simulink model "lr4"  (R2022a)
settings: Solver=FixedStepAuto  StartTime=0.0  StopTime=inf  FixedStep=1e-2  RelTol=1e-3
libraries: instrumentseriallib x3
settings Model: Creator=User  LastModifiedBy=User

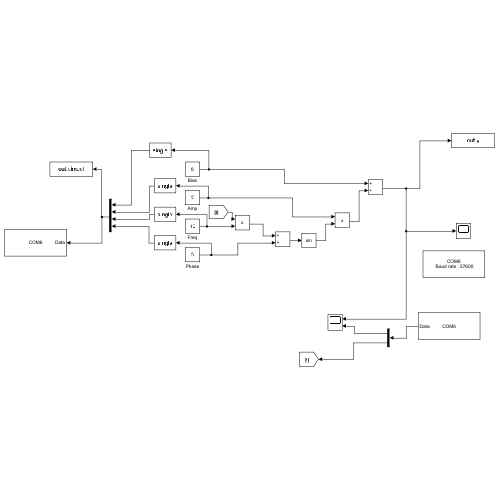
[thumbnail: Simulink's stored preview of the top-level diagram]
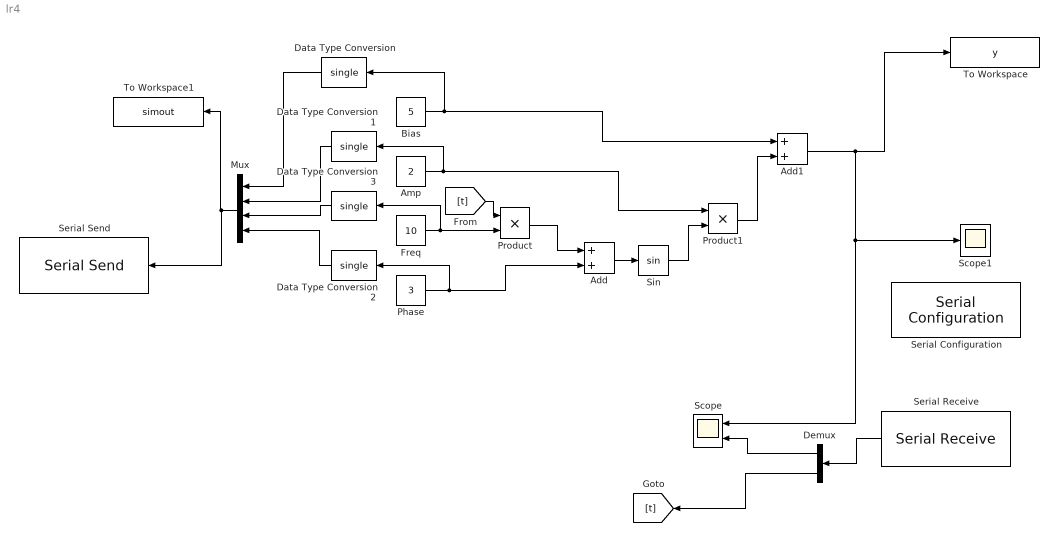
== system lr4 ==
  Add : Sum
  Add1 : Sum
  Amp : Constant  Value=2  OutDataTypeStr=int8
  Bias : Constant  Value=5  OutDataTypeStr=int8
  Data Type Conversion{,1..3} (4 alike) : DataTypeConversion  OutDataTypeStr=single  SaturateOnIntegerOverflow=off  RndMeth=Floor
  Demux : Demux  Outputs=2
  Freq : Constant  Value=10  OutDataTypeStr=int8
  Mux : Mux
  Phase : Constant  Value=3  OutDataTypeStr=int8
  Product : Product
  Product1 : Product
  Scope : Scope  NumInputPorts=2
  Scope1 : Scope
  Serial Configuration : instrumentseriallib/Serial Configuration  Priority=-200000  PortSel=COM6  Port=COM6  ComPort=COM6  BaudRate=57600  DataBits=8  Parity=none  StopBits=1  ByteOrder=little-endian  FlowControl=none  Timeout=10  SimulateUsing=Interpreted execution  BlockInModel=on  aMode=1
      settings: SourceProductBaseCode=OT,IC,MT
  Serial Receive : instrumentseriallib/Serial Receive  Priority=1  PortSel=COM6  Port=COM6  ComPort=COM6  DataType=single  SaveDataType=uint8  ToggleHeader=on  Header='rrrr'  ToggleTerminator=on  Terminator=Custom terminator  CustomTerminator='nnnn'  InputFormat=Row major  ToggleDataSize=on  DataSize=[1 2]  EnableBlockingMode=on  ActionDataUnavailable=Output custom value  ActionWhenDataUnavailable=Output custom value  CustomValue=-1  SampleTime=0.01  SimulateUsing=Interpreted execution  BlockInModel=on  aMode=1
      settings: SourceProductBaseCode=OT,IC,MT
  Serial Send : instrumentseriallib/Serial Send  Priority=1  PortSel=COM6  Port=COM6  ComPort=COM6  Header='rrrr'  Terminator=Custom terminator  CustomTerminator='nnnn'  EnableBlockingMode=on  SimulateUsing=Interpreted execution  BlockInModel=on  aMode=1
      settings: SourceProductBaseCode=OT,IC,MT
  Sin : Trigonometry
  To Workspace : ToWorkspace  VariableName=y  SaveFormat=Timeseries  SampleTime=-1
  To Workspace1 : ToWorkspace  VariableName=simout  SaveFormat=Timeseries  SampleTime=-1
  wires:
  [t] -> Product/1
  Freq/1 -> Data Type Conversion3/1, Product/2
  Product/1 -> Add/1
  Add/1 -> Sin/1
  Sin/1 -> Product1/2
  Amp/1 -> Data Type Conversion1/1, Product1/1
  Product1/1 -> Add1/2
  Bias/1 -> Data Type Conversion/1, Add1/1
  Add1/1 -> Scope/1, Scope1/1, To Workspace/1
  Phase/1 -> Add/2, Data Type Conversion2/1
  Mux/1 -> Serial Send/1, To Workspace1/1
  Data Type Conversion/1 -> Mux/1
  Data Type Conversion1/1 -> Mux/2
  Data Type Conversion2/1 -> Mux/4
  Data Type Conversion3/1 -> Mux/3
  Demux/1 -> Scope/2
  Serial Receive/1 -> Demux/1
  Demux/2 -> [t]
